simulink model "Kinematic_Modeling"  (R2021b)
settings: Solver=VariableStepAuto  StartTime=0.0  StopTime=10.0  RelTol=1e-3
libraries: simulink_extras x4
settings Model: Creator=Bishoy Zaky  LastModifiedBy=Bishoy Zaky

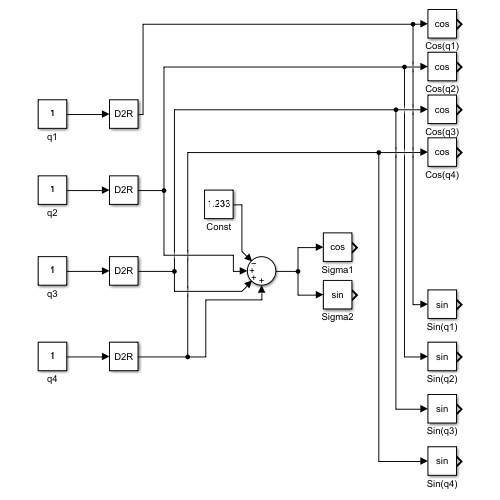
[thumbnail: Simulink's stored preview of the top-level diagram]
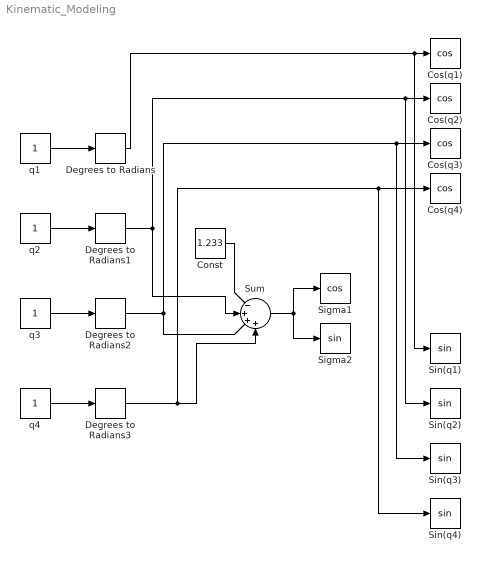
== system Kinematic_Modeling ==
  Const : Constant  Value=1.233
  Cos(q1) : Trigonometry  Operator=cos
  Cos(q2) : Trigonometry  Operator=cos
  Cos(q3) : Trigonometry  Operator=cos
  Cos(q4) : Trigonometry  Operator=cos
  Degrees to Radians{,1..3} (4 alike) : simulink_extras/Transformations/Degrees to Radians
  Sigma1 : Trigonometry  Operator=cos
  Sigma2 : Trigonometry
  Sin(q1) : Trigonometry
  Sin(q2) : Trigonometry
  Sin(q3) : Trigonometry
  Sin(q4) : Trigonometry
  Sum : Sum  Inputs=|-+++
  q{1..4} (4 alike) : Constant
  wires:
  q2/1 -> Degrees to Radians1/1
  q1/1 -> Degrees to Radians/1
  q3/1 -> Degrees to Radians2/1
  q4/1 -> Degrees to Radians3/1
  Degrees to Radians1/1 -> Sin(q2)/1, Cos(q2)/1, Sum/2
  Degrees to Radians2/1 -> Sin(q3)/1, Cos(q3)/1, Sum/3
  Degrees to Radians3/1 -> Sin(q4)/1, Cos(q4)/1, Sum/4
  Const/1 -> Sum/1
  Sum/1 -> Sigma2/1, Sigma1/1
  Degrees to Radians/1 -> Sin(q1)/1, Cos(q1)/1
